simulink model "TST_EngPrt_PrtLimOvht"  (R2016b)
settings: Solver=FixedStepDiscrete  StartTime=0.0  StopTime=0.02  FixedStep=sampleTime  RelTol=1e-3
values from neighbouring files (symbols this model uses):
  testCase = 1    [initTST_EngPrt_PrtLimOvht_001.m]    (also in initTST_EngPrt_PrtLimOvht_002.m = 2; initTST_EngPrt_PrtLimOvht_003.m = 3; initTST_EngPrt_PrtLimOvht_004.m = 4; initTST_EngPrt_PrtLimOvht_005.m = 5)
libraries: simulink x21, UnitTest_Lib x10
(part 2 of 2)

== system TST_EngPrt_PrtLimOvht/simulationInput/testSignals_R003 ==
  BC : BusCreator  Inputs=14
  spec_AFS_mAirPerCyl : FromWorkspace  VariableName=testSig_AFS_mAirPerCyl  Interpolate=off  OutputAfterFinalValue=Holding final value
  spec_Air_tAFS_mp : FromWorkspace  VariableName=testSig_Air_tAFS_mp  Interpolate=off  OutputAfterFinalValue=Holding final value
  spec_Air_tCACDs_mp : FromWorkspace  VariableName=testSig_Air_tCACDs_mp  Interpolate=off  OutputAfterFinalValue=Holding final value
  spec_Air_tIntkVUs : FromWorkspace  VariableName=testSig_Air_tIntkVUs  Interpolate=off  OutputAfterFinalValue=Holding final value
  spec_CEngDsT_t : FromWorkspace  VariableName=testSig_CEngDsT_t  Interpolate=off  OutputAfterFinalValue=Holding final value
  spec_CnvSet_etaCurr : FromWorkspace  VariableName=testSig_CnvSet_etaCurr  Interpolate=off  OutputAfterFinalValue=Holding final value
  spec_DSM_bEngPrtOvhtPrv : FromWorkspace  VariableName=testSig_DSM_bEngPrtOvhtPrv  Interpolate=off  OutputAfterFinalValue=Holding final value
  spec_EngPrt_trqLimOvhtPrv : FromWorkspace  VariableName=testSig_EngPrt_trqLimOvhtPrv  Interpolate=off  OutputAfterFinalValue=Holding final value
  spec_EnvT_t : FromWorkspace  VariableName=testSig_EnvT_t  Interpolate=off  OutputAfterFinalValue=Holding final value
  spec_Epm_nEng : FromWorkspace  VariableName=testSig_Epm_nEng  Interpolate=off  OutputAfterFinalValue=Holding final value
  spec_FuelT_t : FromWorkspace  VariableName=testSig_FuelT_t  Interpolate=off  OutputAfterFinalValue=Holding final value
  spec_InjCtl_qSetUnBal : FromWorkspace  VariableName=testSig_InjCtl_qSetUnBal  Interpolate=off  OutputAfterFinalValue=Holding final value
  spec_Oil_tSwmp : FromWorkspace  VariableName=testSig_Oil_tSwmp  Interpolate=off  OutputAfterFinalValue=Holding final value
  spec_VehV_v : FromWorkspace  VariableName=testSig_VehV_v  Interpolate=off  OutputAfterFinalValue=Holding final value
  testSignals : Outport
  wires:
  BC/1 -> testSignals/1
  spec_Epm_nEng/1 -> BC/1  "testSig_Epm_nEng"
  spec_AFS_mAirPerCyl/1 -> BC/2  "testSig_AFS_mAirPerCyl"
  spec_InjCtl_qSetUnBal/1 -> BC/3  "testSig_InjCtl_qSetUnBal"
  spec_Oil_tSwmp/1 -> BC/4  "testSig_Oil_tSwmp"
  spec_CEngDsT_t/1 -> BC/5  "testSig_CEngDsT_t"
  spec_FuelT_t/1 -> BC/6  "testSig_FuelT_t"
  spec_VehV_v/1 -> BC/7  "testSig_VehV_v"
  spec_CnvSet_etaCurr/1 -> BC/8  "testSig_CnvSet_etaCurr"
  spec_DSM_bEngPrtOvhtPrv/1 -> BC/9  "testSig_DSM_bEngPrtOvhtPrv"
  spec_Air_tCACDs_mp/1 -> BC/10  "testSig_Air_tCACDs_mp"
  spec_Air_tAFS_mp/1 -> BC/11  "testSig_Air_tAFS_mp"
  spec_EnvT_t/1 -> BC/12  "testSig_EnvT_t"
  spec_Air_tIntkVUs/1 -> BC/13  "testSig_Air_tIntkVUs"
  spec_EngPrt_trqLimOvhtPrv/1 -> BC/14  "testSig_EngPrt_trqLimOvhtPrv"

== system TST_EngPrt_PrtLimOvht/simulationInput/testSignals_R004 ==
  BC : BusCreator  Inputs=14
  spec_AFS_mAirPerCyl : FromWorkspace  VariableName=testSig_AFS_mAirPerCyl  Interpolate=off  OutputAfterFinalValue=Holding final value
  spec_Air_tAFS_mp : FromWorkspace  VariableName=testSig_Air_tAFS_mp  Interpolate=off  OutputAfterFinalValue=Holding final value
  spec_Air_tCACDs_mp : FromWorkspace  VariableName=testSig_Air_tCACDs_mp  Interpolate=off  OutputAfterFinalValue=Holding final value
  spec_Air_tIntkVUs : FromWorkspace  VariableName=testSig_Air_tIntkVUs  Interpolate=off  OutputAfterFinalValue=Holding final value
  spec_CEngDsT_t : FromWorkspace  VariableName=testSig_CEngDsT_t  Interpolate=off  OutputAfterFinalValue=Holding final value
  spec_CnvSet_etaCurr : FromWorkspace  VariableName=testSig_CnvSet_etaCurr  Interpolate=off  OutputAfterFinalValue=Holding final value
  spec_DSM_bEngPrtOvhtPrv : FromWorkspace  VariableName=testSig_DSM_bEngPrtOvhtPrv  Interpolate=off  OutputAfterFinalValue=Holding final value
  spec_EngPrt_trqLimOvhtPrv : FromWorkspace  VariableName=testSig_EngPrt_trqLimOvhtPrv  Interpolate=off  OutputAfterFinalValue=Holding final value
  spec_EnvT_t : FromWorkspace  VariableName=testSig_EnvT_t  Interpolate=off  OutputAfterFinalValue=Holding final value
  spec_Epm_nEng : FromWorkspace  VariableName=testSig_Epm_nEng  Interpolate=off  OutputAfterFinalValue=Holding final value
  spec_FuelT_t : FromWorkspace  VariableName=testSig_FuelT_t  Interpolate=off  OutputAfterFinalValue=Holding final value
  spec_InjCtl_qSetUnBal : FromWorkspace  VariableName=testSig_InjCtl_qSetUnBal  Interpolate=off  OutputAfterFinalValue=Holding final value
  spec_Oil_tSwmp : FromWorkspace  VariableName=testSig_Oil_tSwmp  Interpolate=off  OutputAfterFinalValue=Holding final value
  spec_VehV_v : FromWorkspace  VariableName=testSig_VehV_v  Interpolate=off  OutputAfterFinalValue=Holding final value
  testSignals : Outport
  wires:
  BC/1 -> testSignals/1
  spec_Epm_nEng/1 -> BC/1  "testSig_Epm_nEng"
  spec_AFS_mAirPerCyl/1 -> BC/2  "testSig_AFS_mAirPerCyl"
  spec_InjCtl_qSetUnBal/1 -> BC/3  "testSig_InjCtl_qSetUnBal"
  spec_Oil_tSwmp/1 -> BC/4  "testSig_Oil_tSwmp"
  spec_CEngDsT_t/1 -> BC/5  "testSig_CEngDsT_t"
  spec_FuelT_t/1 -> BC/6  "testSig_FuelT_t"
  spec_VehV_v/1 -> BC/7  "testSig_VehV_v"
  spec_CnvSet_etaCurr/1 -> BC/8  "testSig_CnvSet_etaCurr"
  spec_DSM_bEngPrtOvhtPrv/1 -> BC/9  "testSig_DSM_bEngPrtOvhtPrv"
  spec_Air_tCACDs_mp/1 -> BC/10  "testSig_Air_tCACDs_mp"
  spec_Air_tAFS_mp/1 -> BC/11  "testSig_Air_tAFS_mp"
  spec_EnvT_t/1 -> BC/12  "testSig_EnvT_t"
  spec_Air_tIntkVUs/1 -> BC/13  "testSig_Air_tIntkVUs"
  spec_EngPrt_trqLimOvhtPrv/1 -> BC/14  "testSig_EngPrt_trqLimOvhtPrv"

== system TST_EngPrt_PrtLimOvht/simulationInput/testSignals_R005 ==
  BC : BusCreator  Inputs=14
  spec_AFS_mAirPerCyl : FromWorkspace  VariableName=testSig_AFS_mAirPerCyl  Interpolate=off  OutputAfterFinalValue=Holding final value
  spec_Air_tAFS_mp : FromWorkspace  VariableName=testSig_Air_tAFS_mp  Interpolate=off  OutputAfterFinalValue=Holding final value
  spec_Air_tCACDs_mp : FromWorkspace  VariableName=testSig_Air_tCACDs_mp  Interpolate=off  OutputAfterFinalValue=Holding final value
  spec_Air_tIntkVUs : FromWorkspace  VariableName=testSig_Air_tIntkVUs  Interpolate=off  OutputAfterFinalValue=Holding final value
  spec_CEngDsT_t : FromWorkspace  VariableName=testSig_CEngDsT_t  Interpolate=off  OutputAfterFinalValue=Holding final value
  spec_CnvSet_etaCurr : FromWorkspace  VariableName=testSig_CnvSet_etaCurr  Interpolate=off  OutputAfterFinalValue=Holding final value
  spec_DSM_bEngPrtOvhtPrv : FromWorkspace  VariableName=testSig_DSM_bEngPrtOvhtPrv  Interpolate=off  OutputAfterFinalValue=Holding final value
  spec_EngPrt_trqLimOvhtPrv : FromWorkspace  VariableName=testSig_EngPrt_trqLimOvhtPrv  Interpolate=off  OutputAfterFinalValue=Holding final value
  spec_EnvT_t : FromWorkspace  VariableName=testSig_EnvT_t  Interpolate=off  OutputAfterFinalValue=Holding final value
  spec_Epm_nEng : FromWorkspace  VariableName=testSig_Epm_nEng  Interpolate=off  OutputAfterFinalValue=Holding final value
  spec_FuelT_t : FromWorkspace  VariableName=testSig_FuelT_t  Interpolate=off  OutputAfterFinalValue=Holding final value
  spec_InjCtl_qSetUnBal : FromWorkspace  VariableName=testSig_InjCtl_qSetUnBal  Interpolate=off  OutputAfterFinalValue=Holding final value
  spec_Oil_tSwmp : FromWorkspace  VariableName=testSig_Oil_tSwmp  Interpolate=off  OutputAfterFinalValue=Holding final value
  spec_VehV_v : FromWorkspace  VariableName=testSig_VehV_v  Interpolate=off  OutputAfterFinalValue=Holding final value
  testSignals : Outport
  wires:
  BC/1 -> testSignals/1
  spec_Epm_nEng/1 -> BC/1  "testSig_Epm_nEng"
  spec_AFS_mAirPerCyl/1 -> BC/2  "testSig_AFS_mAirPerCyl"
  spec_InjCtl_qSetUnBal/1 -> BC/3  "testSig_InjCtl_qSetUnBal"
  spec_Oil_tSwmp/1 -> BC/4  "testSig_Oil_tSwmp"
  spec_CEngDsT_t/1 -> BC/5  "testSig_CEngDsT_t"
  spec_FuelT_t/1 -> BC/6  "testSig_FuelT_t"
  spec_VehV_v/1 -> BC/7  "testSig_VehV_v"
  spec_CnvSet_etaCurr/1 -> BC/8  "testSig_CnvSet_etaCurr"
  spec_DSM_bEngPrtOvhtPrv/1 -> BC/9  "testSig_DSM_bEngPrtOvhtPrv"
  spec_Air_tCACDs_mp/1 -> BC/10  "testSig_Air_tCACDs_mp"
  spec_Air_tAFS_mp/1 -> BC/11  "testSig_Air_tAFS_mp"
  spec_EnvT_t/1 -> BC/12  "testSig_EnvT_t"
  spec_Air_tIntkVUs/1 -> BC/13  "testSig_Air_tIntkVUs"
  spec_EngPrt_trqLimOvhtPrv/1 -> BC/14  "testSig_EngPrt_trqLimOvhtPrv"

== system TST_EngPrt_PrtLimOvht/simulationInput/testSignals_R006 ==
  BC : BusCreator  Inputs=14
  spec_AFS_mAirPerCyl : FromWorkspace  VariableName=testSig_AFS_mAirPerCyl  Interpolate=off  OutputAfterFinalValue=Holding final value
  spec_Air_tAFS_mp : FromWorkspace  VariableName=testSig_Air_tAFS_mp  Interpolate=off  OutputAfterFinalValue=Holding final value
  spec_Air_tCACDs_mp : FromWorkspace  VariableName=testSig_Air_tCACDs_mp  Interpolate=off  OutputAfterFinalValue=Holding final value
  spec_Air_tIntkVUs : FromWorkspace  VariableName=testSig_Air_tIntkVUs  Interpolate=off  OutputAfterFinalValue=Holding final value
  spec_CEngDsT_t : FromWorkspace  VariableName=testSig_CEngDsT_t  Interpolate=off  OutputAfterFinalValue=Holding final value
  spec_CnvSet_etaCurr : FromWorkspace  VariableName=testSig_CnvSet_etaCurr  Interpolate=off  OutputAfterFinalValue=Holding final value
  spec_DSM_bEngPrtOvhtPrv : FromWorkspace  VariableName=testSig_DSM_bEngPrtOvhtPrv  Interpolate=off  OutputAfterFinalValue=Holding final value
  spec_EngPrt_trqLimOvhtPrv : FromWorkspace  VariableName=testSig_EngPrt_trqLimOvhtPrv  Interpolate=off  OutputAfterFinalValue=Holding final value
  spec_EnvT_t : FromWorkspace  VariableName=testSig_EnvT_t  Interpolate=off  OutputAfterFinalValue=Holding final value
  spec_Epm_nEng : FromWorkspace  VariableName=testSig_Epm_nEng  Interpolate=off  OutputAfterFinalValue=Holding final value
  spec_FuelT_t : FromWorkspace  VariableName=testSig_FuelT_t  Interpolate=off  OutputAfterFinalValue=Holding final value
  spec_InjCtl_qSetUnBal : FromWorkspace  VariableName=testSig_InjCtl_qSetUnBal  Interpolate=off  OutputAfterFinalValue=Holding final value
  spec_Oil_tSwmp : FromWorkspace  VariableName=testSig_Oil_tSwmp  Interpolate=off  OutputAfterFinalValue=Holding final value
  spec_VehV_v : FromWorkspace  VariableName=testSig_VehV_v  Interpolate=off  OutputAfterFinalValue=Holding final value
  testSignals : Outport
  wires:
  BC/1 -> testSignals/1
  spec_Epm_nEng/1 -> BC/1  "testSig_Epm_nEng"
  spec_AFS_mAirPerCyl/1 -> BC/2  "testSig_AFS_mAirPerCyl"
  spec_InjCtl_qSetUnBal/1 -> BC/3  "testSig_InjCtl_qSetUnBal"
  spec_Oil_tSwmp/1 -> BC/4  "testSig_Oil_tSwmp"
  spec_CEngDsT_t/1 -> BC/5  "testSig_CEngDsT_t"
  spec_FuelT_t/1 -> BC/6  "testSig_FuelT_t"
  spec_VehV_v/1 -> BC/7  "testSig_VehV_v"
  spec_CnvSet_etaCurr/1 -> BC/8  "testSig_CnvSet_etaCurr"
  spec_DSM_bEngPrtOvhtPrv/1 -> BC/9  "testSig_DSM_bEngPrtOvhtPrv"
  spec_Air_tCACDs_mp/1 -> BC/10  "testSig_Air_tCACDs_mp"
  spec_Air_tAFS_mp/1 -> BC/11  "testSig_Air_tAFS_mp"
  spec_EnvT_t/1 -> BC/12  "testSig_EnvT_t"
  spec_Air_tIntkVUs/1 -> BC/13  "testSig_Air_tIntkVUs"
  spec_EngPrt_trqLimOvhtPrv/1 -> BC/14  "testSig_EngPrt_trqLimOvhtPrv"

== system TST_EngPrt_PrtLimOvht/simulationInput/testSignals_R007 ==
  BC : BusCreator  Inputs=14
  spec_AFS_mAirPerCyl : FromWorkspace  VariableName=testSig_AFS_mAirPerCyl  Interpolate=off  OutputAfterFinalValue=Holding final value
  spec_Air_tAFS_mp : FromWorkspace  VariableName=testSig_Air_tAFS_mp  Interpolate=off  OutputAfterFinalValue=Holding final value
  spec_Air_tCACDs_mp : FromWorkspace  VariableName=testSig_Air_tCACDs_mp  Interpolate=off  OutputAfterFinalValue=Holding final value
  spec_Air_tIntkVUs : FromWorkspace  VariableName=testSig_Air_tIntkVUs  Interpolate=off  OutputAfterFinalValue=Holding final value
  spec_CEngDsT_t : FromWorkspace  VariableName=testSig_CEngDsT_t  Interpolate=off  OutputAfterFinalValue=Holding final value
  spec_CnvSet_etaCurr : FromWorkspace  VariableName=testSig_CnvSet_etaCurr  Interpolate=off  OutputAfterFinalValue=Holding final value
  spec_DSM_bEngPrtOvhtPrv : FromWorkspace  VariableName=testSig_DSM_bEngPrtOvhtPrv  Interpolate=off  OutputAfterFinalValue=Holding final value
  spec_EngPrt_trqLimOvhtPrv : FromWorkspace  VariableName=testSig_EngPrt_trqLimOvhtPrv  Interpolate=off  OutputAfterFinalValue=Holding final value
  spec_EnvT_t : FromWorkspace  VariableName=testSig_EnvT_t  Interpolate=off  OutputAfterFinalValue=Holding final value
  spec_Epm_nEng : FromWorkspace  VariableName=testSig_Epm_nEng  Interpolate=off  OutputAfterFinalValue=Holding final value
  spec_FuelT_t : FromWorkspace  VariableName=testSig_FuelT_t  Interpolate=off  OutputAfterFinalValue=Holding final value
  spec_InjCtl_qSetUnBal : FromWorkspace  VariableName=testSig_InjCtl_qSetUnBal  Interpolate=off  OutputAfterFinalValue=Holding final value
  spec_Oil_tSwmp : FromWorkspace  VariableName=testSig_Oil_tSwmp  Interpolate=off  OutputAfterFinalValue=Holding final value
  spec_VehV_v : FromWorkspace  VariableName=testSig_VehV_v  Interpolate=off  OutputAfterFinalValue=Holding final value
  testSignals : Outport
  wires:
  BC/1 -> testSignals/1
  spec_Epm_nEng/1 -> BC/1  "testSig_Epm_nEng"
  spec_AFS_mAirPerCyl/1 -> BC/2  "testSig_AFS_mAirPerCyl"
  spec_InjCtl_qSetUnBal/1 -> BC/3  "testSig_InjCtl_qSetUnBal"
  spec_Oil_tSwmp/1 -> BC/4  "testSig_Oil_tSwmp"
  spec_CEngDsT_t/1 -> BC/5  "testSig_CEngDsT_t"
  spec_FuelT_t/1 -> BC/6  "testSig_FuelT_t"
  spec_VehV_v/1 -> BC/7  "testSig_VehV_v"
  spec_CnvSet_etaCurr/1 -> BC/8  "testSig_CnvSet_etaCurr"
  spec_DSM_bEngPrtOvhtPrv/1 -> BC/9  "testSig_DSM_bEngPrtOvhtPrv"
  spec_Air_tCACDs_mp/1 -> BC/10  "testSig_Air_tCACDs_mp"
  spec_Air_tAFS_mp/1 -> BC/11  "testSig_Air_tAFS_mp"
  spec_EnvT_t/1 -> BC/12  "testSig_EnvT_t"
  spec_Air_tIntkVUs/1 -> BC/13  "testSig_Air_tIntkVUs"
  spec_EngPrt_trqLimOvhtPrv/1 -> BC/14  "testSig_EngPrt_trqLimOvhtPrv"

== system TST_EngPrt_PrtLimOvht/simulationInput/testSignals_R008 ==
  BC : BusCreator  Inputs=14
  spec_AFS_mAirPerCyl : FromWorkspace  VariableName=testSig_AFS_mAirPerCyl  Interpolate=off  OutputAfterFinalValue=Holding final value
  spec_Air_tAFS_mp : FromWorkspace  VariableName=testSig_Air_tAFS_mp  Interpolate=off  OutputAfterFinalValue=Holding final value
  spec_Air_tCACDs_mp : FromWorkspace  VariableName=testSig_Air_tCACDs_mp  Interpolate=off  OutputAfterFinalValue=Holding final value
  spec_Air_tIntkVUs : FromWorkspace  VariableName=testSig_Air_tIntkVUs  Interpolate=off  OutputAfterFinalValue=Holding final value
  spec_CEngDsT_t : FromWorkspace  VariableName=testSig_CEngDsT_t  Interpolate=off  OutputAfterFinalValue=Holding final value
  spec_CnvSet_etaCurr : FromWorkspace  VariableName=testSig_CnvSet_etaCurr  Interpolate=off  OutputAfterFinalValue=Holding final value
  spec_DSM_bEngPrtOvhtPrv : FromWorkspace  VariableName=testSig_DSM_bEngPrtOvhtPrv  Interpolate=off  OutputAfterFinalValue=Holding final value
  spec_EngPrt_trqLimOvhtPrv : FromWorkspace  VariableName=testSig_EngPrt_trqLimOvhtPrv  Interpolate=off  OutputAfterFinalValue=Holding final value
  spec_EnvT_t : FromWorkspace  VariableName=testSig_EnvT_t  Interpolate=off  OutputAfterFinalValue=Holding final value
  spec_Epm_nEng : FromWorkspace  VariableName=testSig_Epm_nEng  Interpolate=off  OutputAfterFinalValue=Holding final value
  spec_FuelT_t : FromWorkspace  VariableName=testSig_FuelT_t  Interpolate=off  OutputAfterFinalValue=Holding final value
  spec_InjCtl_qSetUnBal : FromWorkspace  VariableName=testSig_InjCtl_qSetUnBal  Interpolate=off  OutputAfterFinalValue=Holding final value
  spec_Oil_tSwmp : FromWorkspace  VariableName=testSig_Oil_tSwmp  Interpolate=off  OutputAfterFinalValue=Holding final value
  spec_VehV_v : FromWorkspace  VariableName=testSig_VehV_v  Interpolate=off  OutputAfterFinalValue=Holding final value
  testSignals : Outport
  wires:
  BC/1 -> testSignals/1
  spec_Epm_nEng/1 -> BC/1  "testSig_Epm_nEng"
  spec_AFS_mAirPerCyl/1 -> BC/2  "testSig_AFS_mAirPerCyl"
  spec_InjCtl_qSetUnBal/1 -> BC/3  "testSig_InjCtl_qSetUnBal"
  spec_Oil_tSwmp/1 -> BC/4  "testSig_Oil_tSwmp"
  spec_CEngDsT_t/1 -> BC/5  "testSig_CEngDsT_t"
  spec_FuelT_t/1 -> BC/6  "testSig_FuelT_t"
  spec_VehV_v/1 -> BC/7  "testSig_VehV_v"
  spec_CnvSet_etaCurr/1 -> BC/8  "testSig_CnvSet_etaCurr"
  spec_DSM_bEngPrtOvhtPrv/1 -> BC/9  "testSig_DSM_bEngPrtOvhtPrv"
  spec_Air_tCACDs_mp/1 -> BC/10  "testSig_Air_tCACDs_mp"
  spec_Air_tAFS_mp/1 -> BC/11  "testSig_Air_tAFS_mp"
  spec_EnvT_t/1 -> BC/12  "testSig_EnvT_t"
  spec_Air_tIntkVUs/1 -> BC/13  "testSig_Air_tIntkVUs"
  spec_EngPrt_trqLimOvhtPrv/1 -> BC/14  "testSig_EngPrt_trqLimOvhtPrv"

== system TST_EngPrt_PrtLimOvht/simulationInput/testSignals_R009 ==
  BC : BusCreator  Inputs=14
  spec_AFS_mAirPerCyl : FromWorkspace  VariableName=testSig_AFS_mAirPerCyl  Interpolate=off  OutputAfterFinalValue=Holding final value
  spec_Air_tAFS_mp : FromWorkspace  VariableName=testSig_Air_tAFS_mp  Interpolate=off  OutputAfterFinalValue=Holding final value
  spec_Air_tCACDs_mp : FromWorkspace  VariableName=testSig_Air_tCACDs_mp  Interpolate=off  OutputAfterFinalValue=Holding final value
  spec_Air_tIntkVUs : FromWorkspace  VariableName=testSig_Air_tIntkVUs  Interpolate=off  OutputAfterFinalValue=Holding final value
  spec_CEngDsT_t : FromWorkspace  VariableName=testSig_CEngDsT_t  Interpolate=off  OutputAfterFinalValue=Holding final value
  spec_CnvSet_etaCurr : FromWorkspace  VariableName=testSig_CnvSet_etaCurr  Interpolate=off  OutputAfterFinalValue=Holding final value
  spec_DSM_bEngPrtOvhtPrv : FromWorkspace  VariableName=testSig_DSM_bEngPrtOvhtPrv  Interpolate=off  OutputAfterFinalValue=Holding final value
  spec_EngPrt_trqLimOvhtPrv : FromWorkspace  VariableName=testSig_EngPrt_trqLimOvhtPrv  Interpolate=off  OutputAfterFinalValue=Holding final value
  spec_EnvT_t : FromWorkspace  VariableName=testSig_EnvT_t  Interpolate=off  OutputAfterFinalValue=Holding final value
  spec_Epm_nEng : FromWorkspace  VariableName=testSig_Epm_nEng  Interpolate=off  OutputAfterFinalValue=Holding final value
  spec_FuelT_t : FromWorkspace  VariableName=testSig_FuelT_t  Interpolate=off  OutputAfterFinalValue=Holding final value
  spec_InjCtl_qSetUnBal : FromWorkspace  VariableName=testSig_InjCtl_qSetUnBal  Interpolate=off  OutputAfterFinalValue=Holding final value
  spec_Oil_tSwmp : FromWorkspace  VariableName=testSig_Oil_tSwmp  Interpolate=off  OutputAfterFinalValue=Holding final value
  spec_VehV_v : FromWorkspace  VariableName=testSig_VehV_v  Interpolate=off  OutputAfterFinalValue=Holding final value
  testSignals : Outport
  wires:
  BC/1 -> testSignals/1
  spec_Epm_nEng/1 -> BC/1  "testSig_Epm_nEng"
  spec_AFS_mAirPerCyl/1 -> BC/2  "testSig_AFS_mAirPerCyl"
  spec_InjCtl_qSetUnBal/1 -> BC/3  "testSig_InjCtl_qSetUnBal"
  spec_Oil_tSwmp/1 -> BC/4  "testSig_Oil_tSwmp"
  spec_CEngDsT_t/1 -> BC/5  "testSig_CEngDsT_t"
  spec_FuelT_t/1 -> BC/6  "testSig_FuelT_t"
  spec_VehV_v/1 -> BC/7  "testSig_VehV_v"
  spec_CnvSet_etaCurr/1 -> BC/8  "testSig_CnvSet_etaCurr"
  spec_DSM_bEngPrtOvhtPrv/1 -> BC/9  "testSig_DSM_bEngPrtOvhtPrv"
  spec_Air_tCACDs_mp/1 -> BC/10  "testSig_Air_tCACDs_mp"
  spec_Air_tAFS_mp/1 -> BC/11  "testSig_Air_tAFS_mp"
  spec_EnvT_t/1 -> BC/12  "testSig_EnvT_t"
  spec_Air_tIntkVUs/1 -> BC/13  "testSig_Air_tIntkVUs"
  spec_EngPrt_trqLimOvhtPrv/1 -> BC/14  "testSig_EngPrt_trqLimOvhtPrv"

== system TST_EngPrt_PrtLimOvht/simulationInput/testSignals_R010 ==
  BC : BusCreator  Inputs=14
  spec_AFS_mAirPerCyl : FromWorkspace  VariableName=testSig_AFS_mAirPerCyl  Interpolate=off  OutputAfterFinalValue=Holding final value
  spec_Air_tAFS_mp : FromWorkspace  VariableName=testSig_Air_tAFS_mp  Interpolate=off  OutputAfterFinalValue=Holding final value
  spec_Air_tCACDs_mp : FromWorkspace  VariableName=testSig_Air_tCACDs_mp  Interpolate=off  OutputAfterFinalValue=Holding final value
  spec_Air_tIntkVUs : FromWorkspace  VariableName=testSig_Air_tIntkVUs  Interpolate=off  OutputAfterFinalValue=Holding final value
  spec_CEngDsT_t : FromWorkspace  VariableName=testSig_CEngDsT_t  Interpolate=off  OutputAfterFinalValue=Holding final value
  spec_CnvSet_etaCurr : FromWorkspace  VariableName=testSig_CnvSet_etaCurr  Interpolate=off  OutputAfterFinalValue=Holding final value
  spec_DSM_bEngPrtOvhtPrv : FromWorkspace  VariableName=testSig_DSM_bEngPrtOvhtPrv  Interpolate=off  OutputAfterFinalValue=Holding final value
  spec_EngPrt_trqLimOvhtPrv : FromWorkspace  VariableName=testSig_EngPrt_trqLimOvhtPrv  Interpolate=off  OutputAfterFinalValue=Holding final value
  spec_EnvT_t : FromWorkspace  VariableName=testSig_EnvT_t  Interpolate=off  OutputAfterFinalValue=Holding final value
  spec_Epm_nEng : FromWorkspace  VariableName=testSig_Epm_nEng  Interpolate=off  OutputAfterFinalValue=Holding final value
  spec_FuelT_t : FromWorkspace  VariableName=testSig_FuelT_t  Interpolate=off  OutputAfterFinalValue=Holding final value
  spec_InjCtl_qSetUnBal : FromWorkspace  VariableName=testSig_InjCtl_qSetUnBal  Interpolate=off  OutputAfterFinalValue=Holding final value
  spec_Oil_tSwmp : FromWorkspace  VariableName=testSig_Oil_tSwmp  Interpolate=off  OutputAfterFinalValue=Holding final value
  spec_VehV_v : FromWorkspace  VariableName=testSig_VehV_v  Interpolate=off  OutputAfterFinalValue=Holding final value
  testSignals : Outport
  wires:
  BC/1 -> testSignals/1
  spec_Epm_nEng/1 -> BC/1  "testSig_Epm_nEng"
  spec_AFS_mAirPerCyl/1 -> BC/2  "testSig_AFS_mAirPerCyl"
  spec_InjCtl_qSetUnBal/1 -> BC/3  "testSig_InjCtl_qSetUnBal"
  spec_Oil_tSwmp/1 -> BC/4  "testSig_Oil_tSwmp"
  spec_CEngDsT_t/1 -> BC/5  "testSig_CEngDsT_t"
  spec_FuelT_t/1 -> BC/6  "testSig_FuelT_t"
  spec_VehV_v/1 -> BC/7  "testSig_VehV_v"
  spec_CnvSet_etaCurr/1 -> BC/8  "testSig_CnvSet_etaCurr"
  spec_DSM_bEngPrtOvhtPrv/1 -> BC/9  "testSig_DSM_bEngPrtOvhtPrv"
  spec_Air_tCACDs_mp/1 -> BC/10  "testSig_Air_tCACDs_mp"
  spec_Air_tAFS_mp/1 -> BC/11  "testSig_Air_tAFS_mp"
  spec_EnvT_t/1 -> BC/12  "testSig_EnvT_t"
  spec_Air_tIntkVUs/1 -> BC/13  "testSig_Air_tIntkVUs"
  spec_EngPrt_trqLimOvhtPrv/1 -> BC/14  "testSig_EngPrt_trqLimOvhtPrv"

== system TST_EngPrt_PrtLimOvht/compareSignals/Requirement_001/specifyOutputs ==
  sig_Req_Bus : Inport
  sig_Result_Bus : Inport  Port=2
  AndN : Logic  Inputs=1
  BS_Req : BusSelector  OutputSignals=testSig_EngPrt_trqLimOvhtPrv
  BS_Result : BusSelector  OutputSignals=EngPrt_trqLimOvhtPrv
  Bitwise_And1 : simulink/Logic and Bit Operations/Bitwise Operator  logicop=AND  UseBitMask=off  BitMask=bin2dec('11011001')  BitMaskRealWorld=Stored Integer
  Scope : Scope
  Scope1 : Scope  NumInputPorts=2
  cmp_1 : UnitTest_Lib/RoughlyEqual  slope=0.1
  result_tws : ToWorkspace  VariableName=spec_result_001
  tws_1 : ToWorkspace  VariableName=spec_req_001_001
  result : Outport
  wires:
  sig_Req_Bus/1 -> BS_Req/1
  sig_Result_Bus/1 -> BS_Result/1
  AndN/1 -> result/1, result_tws/1
  BS_Req/1 -> cmp_1/1, Scope1/1  "<testSig_EngPrt_trqLimOvhtPrv>"
  BS_Result/1 -> cmp_1/2, Scope1/2  "<EngPrt_trqLimOvhtPrv>"
  cmp_1/1 -> Bitwise_And1/1
  Bitwise_And1/1 -> tws_1/1, AndN/1, Scope/1

== system TST_EngPrt_PrtLimOvht/compareSignals/Requirement_002/specifyOutputs ==
  sig_Req_Bus : Inport
  sig_Result_Bus : Inport  Port=2
  AndN : Logic  Inputs=1
  BS_Req : BusSelector  OutputSignals=testSig_EngPrt_trqLimOvhtPrv
  BS_Result : BusSelector  OutputSignals=EngPrt_trqLimOvhtPrv
  Bitwise_And1 : simulink/Logic and Bit Operations/Bitwise Operator  logicop=AND  UseBitMask=off  BitMask=bin2dec('11011001')  BitMaskRealWorld=Stored Integer
  Scope : Scope
  Scope1 : Scope  NumInputPorts=2
  cmp_1 : UnitTest_Lib/RoughlyEqual  slope=0.1
  result_tws : ToWorkspace  VariableName=spec_result_002
  tws_1 : ToWorkspace  VariableName=spec_req_002_001
  result : Outport
  wires:
  sig_Req_Bus/1 -> BS_Req/1
  sig_Result_Bus/1 -> BS_Result/1
  AndN/1 -> result/1, result_tws/1
  BS_Req/1 -> cmp_1/1, Scope1/1  "<testSig_EngPrt_trqLimOvhtPrv>"
  BS_Result/1 -> cmp_1/2, Scope1/2  "<EngPrt_trqLimOvhtPrv>"
  cmp_1/1 -> Bitwise_And1/1
  Bitwise_And1/1 -> tws_1/1, AndN/1, Scope/1

== system TST_EngPrt_PrtLimOvht/compareSignals/Requirement_003/specifyOutputs ==
  sig_Req_Bus : Inport
  sig_Result_Bus : Inport  Port=2
  AndN : Logic  Inputs=1
  BS_Req : BusSelector  OutputSignals=testSig_EngPrt_trqLimOvhtPrv
  BS_Result : BusSelector  OutputSignals=EngPrt_trqLimOvhtPrv
  Bitwise_And1 : simulink/Logic and Bit Operations/Bitwise Operator  logicop=AND  UseBitMask=off  BitMask=bin2dec('11011001')  BitMaskRealWorld=Stored Integer
  Scope : Scope
  Scope1 : Scope  NumInputPorts=2
  cmp_1 : UnitTest_Lib/RoughlyEqual  slope=0.1
  result_tws : ToWorkspace  VariableName=spec_result_003
  tws_1 : ToWorkspace  VariableName=spec_req_003_001
  result : Outport
  wires:
  sig_Req_Bus/1 -> BS_Req/1
  sig_Result_Bus/1 -> BS_Result/1
  AndN/1 -> result/1, result_tws/1
  BS_Req/1 -> cmp_1/1, Scope1/1  "<testSig_EngPrt_trqLimOvhtPrv>"
  BS_Result/1 -> cmp_1/2, Scope1/2  "<EngPrt_trqLimOvhtPrv>"
  cmp_1/1 -> Bitwise_And1/1
  Bitwise_And1/1 -> AndN/1, Scope/1, tws_1/1

== system TST_EngPrt_PrtLimOvht/compareSignals/Requirement_004/specifyOutputs ==
  sig_Req_Bus : Inport
  sig_Result_Bus : Inport  Port=2
  AndN : Logic  Inputs=1
  BS_Req : BusSelector  OutputSignals=testSig_EngPrt_trqLimOvhtPrv
  BS_Result : BusSelector  OutputSignals=EngPrt_trqLimOvhtPrv
  Bitwise_And1 : simulink/Logic and Bit Operations/Bitwise Operator  logicop=AND  UseBitMask=off  BitMask=bin2dec('11011001')  BitMaskRealWorld=Stored Integer
  Scope : Scope
  Scope1 : Scope  NumInputPorts=2
  cmp_1 : UnitTest_Lib/RoughlyEqual  slope=0.5
  result_tws : ToWorkspace  VariableName=spec_result_004
  tws_1 : ToWorkspace  VariableName=spec_req_004_001
  result : Outport
  wires:
  sig_Req_Bus/1 -> BS_Req/1
  sig_Result_Bus/1 -> BS_Result/1
  AndN/1 -> result/1, result_tws/1
  BS_Req/1 -> cmp_1/1, Scope1/1  "<testSig_EngPrt_trqLimOvhtPrv>"
  BS_Result/1 -> cmp_1/2, Scope1/2  "<EngPrt_trqLimOvhtPrv>"
  cmp_1/1 -> Bitwise_And1/1
  Bitwise_And1/1 -> AndN/1, Scope/1, tws_1/1

== system TST_EngPrt_PrtLimOvht/compareSignals/Requirement_005/specifyOutputs ==
  sig_Req_Bus : Inport
  sig_Result_Bus : Inport  Port=2
  AndN : Logic  Inputs=1
  BS_Req : BusSelector  OutputSignals=testSig_EngPrt_trqLimOvhtPrv
  BS_Result : BusSelector  OutputSignals=EngPrt_trqLimOvhtPrv
  Bitwise_And1 : simulink/Logic and Bit Operations/Bitwise Operator  logicop=AND  UseBitMask=off  BitMask=bin2dec('11011001')  BitMaskRealWorld=Stored Integer
  Scope : Scope
  Scope1 : Scope  NumInputPorts=2
  cmp_1 : UnitTest_Lib/RoughlyEqual  slope=0.5
  result_tws : ToWorkspace  VariableName=spec_result_005
  tws_1 : ToWorkspace  VariableName=spec_req_005_001
  result : Outport
  wires:
  sig_Req_Bus/1 -> BS_Req/1
  sig_Result_Bus/1 -> BS_Result/1
  AndN/1 -> result/1, result_tws/1
  BS_Req/1 -> cmp_1/1, Scope1/1  "<testSig_EngPrt_trqLimOvhtPrv>"
  BS_Result/1 -> cmp_1/2, Scope1/2  "<EngPrt_trqLimOvhtPrv>"
  cmp_1/1 -> Bitwise_And1/1
  Bitwise_And1/1 -> AndN/1, Scope/1, tws_1/1

== system TST_EngPrt_PrtLimOvht/compareSignals/Requirement_006/specifyOutputs ==
  sig_Req_Bus : Inport
  sig_Result_Bus : Inport  Port=2
  AndN : Logic  Inputs=1
  BS_Req : BusSelector  OutputSignals=testSig_EngPrt_trqLimOvhtPrv
  BS_Result : BusSelector  OutputSignals=EngPrt_trqLimOvhtPrv
  Bitwise_And1 : simulink/Logic and Bit Operations/Bitwise Operator  logicop=AND  UseBitMask=off  BitMask=bin2dec('11011001')  BitMaskRealWorld=Stored Integer
  Scope : Scope
  Scope1 : Scope  NumInputPorts=2
  cmp_1 : UnitTest_Lib/RoughlyEqual  slope=0.5
  result_tws : ToWorkspace  VariableName=spec_result_006
  tws_1 : ToWorkspace  VariableName=spec_req_006_001
  result : Outport
  wires:
  sig_Req_Bus/1 -> BS_Req/1
  sig_Result_Bus/1 -> BS_Result/1
  AndN/1 -> result/1, result_tws/1
  BS_Req/1 -> cmp_1/1, Scope1/1  "<testSig_EngPrt_trqLimOvhtPrv>"
  BS_Result/1 -> cmp_1/2, Scope1/2  "<EngPrt_trqLimOvhtPrv>"
  cmp_1/1 -> Bitwise_And1/1
  Bitwise_And1/1 -> AndN/1, Scope/1, tws_1/1

== system TST_EngPrt_PrtLimOvht/compareSignals/Requirement_007/specifyOutputs ==
  sig_Req_Bus : Inport
  sig_Result_Bus : Inport  Port=2
  AndN : Logic  Inputs=1
  BS_Req : BusSelector  OutputSignals=testSig_EngPrt_trqLimOvhtPrv
  BS_Result : BusSelector  OutputSignals=EngPrt_trqLimOvhtPrv
  Bitwise_And1 : simulink/Logic and Bit Operations/Bitwise Operator  logicop=AND  UseBitMask=off  BitMask=bin2dec('11011001')  BitMaskRealWorld=Stored Integer
  Scope : Scope
  Scope1 : Scope  NumInputPorts=2
  cmp_1 : UnitTest_Lib/RoughlyEqual  slope=0.5
  result_tws : ToWorkspace  VariableName=spec_result_007
  tws_1 : ToWorkspace  VariableName=spec_req_007_001
  result : Outport
  wires:
  sig_Req_Bus/1 -> BS_Req/1
  sig_Result_Bus/1 -> BS_Result/1
  AndN/1 -> result/1, result_tws/1
  BS_Req/1 -> cmp_1/1, Scope1/1  "<testSig_EngPrt_trqLimOvhtPrv>"
  BS_Result/1 -> cmp_1/2, Scope1/2  "<EngPrt_trqLimOvhtPrv>"
  cmp_1/1 -> Bitwise_And1/1
  Bitwise_And1/1 -> AndN/1, Scope/1, tws_1/1

== system TST_EngPrt_PrtLimOvht/compareSignals/Requirement_008/specifyOutputs ==
  sig_Req_Bus : Inport
  sig_Result_Bus : Inport  Port=2
  AndN : Logic  Inputs=1
  BS_Req : BusSelector  OutputSignals=testSig_EngPrt_trqLimOvhtPrv
  BS_Result : BusSelector  OutputSignals=EngPrt_trqLimOvhtPrv
  Bitwise_And1 : simulink/Logic and Bit Operations/Bitwise Operator  logicop=AND  UseBitMask=off  BitMask=bin2dec('11011001')  BitMaskRealWorld=Stored Integer
  Scope : Scope
  Scope1 : Scope  NumInputPorts=2
  cmp_1 : UnitTest_Lib/RoughlyEqual  slope=0.1
  result_tws : ToWorkspace  VariableName=spec_result_008
  tws_1 : ToWorkspace  VariableName=spec_req_008_001
  result : Outport
  wires:
  sig_Req_Bus/1 -> BS_Req/1
  sig_Result_Bus/1 -> BS_Result/1
  AndN/1 -> result/1, result_tws/1
  BS_Req/1 -> cmp_1/1, Scope1/1  "<testSig_EngPrt_trqLimOvhtPrv>"
  BS_Result/1 -> cmp_1/2, Scope1/2  "<EngPrt_trqLimOvhtPrv>"
  cmp_1/1 -> Bitwise_And1/1
  Bitwise_And1/1 -> tws_1/1, AndN/1, Scope/1

== system TST_EngPrt_PrtLimOvht/compareSignals/Requirement_009/specifyOutputs ==
  sig_Req_Bus : Inport
  sig_Result_Bus : Inport  Port=2
  AndN : Logic  Inputs=1
  BS_Req : BusSelector  OutputSignals=testSig_EngPrt_trqLimOvhtPrv
  BS_Result : BusSelector  OutputSignals=EngPrt_trqLimOvhtPrv
  Bitwise_And1 : simulink/Logic and Bit Operations/Bitwise Operator  logicop=AND  UseBitMask=off  BitMask=bin2dec('11011001')  BitMaskRealWorld=Stored Integer
  Scope : Scope
  Scope1 : Scope  NumInputPorts=2
  cmp_1 : UnitTest_Lib/RoughlyEqual  slope=0.1
  result_tws : ToWorkspace  VariableName=spec_result_009
  tws_1 : ToWorkspace  VariableName=spec_req_009_001
  result : Outport
  wires:
  sig_Req_Bus/1 -> BS_Req/1
  sig_Result_Bus/1 -> BS_Result/1
  AndN/1 -> result/1, result_tws/1
  BS_Req/1 -> cmp_1/1, Scope1/1  "<testSig_EngPrt_trqLimOvhtPrv>"
  BS_Result/1 -> cmp_1/2, Scope1/2  "<EngPrt_trqLimOvhtPrv>"
  cmp_1/1 -> Bitwise_And1/1
  Bitwise_And1/1 -> tws_1/1, AndN/1, Scope/1

== system TST_EngPrt_PrtLimOvht/compareSignals/Requirement_010/specifyOutputs ==
  sig_Req_Bus : Inport
  sig_Result_Bus : Inport  Port=2
  AndN : Logic  Inputs=1
  BS_Req : BusSelector  OutputSignals=testSig_EngPrt_trqLimOvhtPrv
  BS_Result : BusSelector  OutputSignals=EngPrt_trqLimOvhtPrv
  Bitwise_And1 : simulink/Logic and Bit Operations/Bitwise Operator  logicop=AND  UseBitMask=off  BitMask=bin2dec('11011001')  BitMaskRealWorld=Stored Integer
  Scope : Scope
  Scope1 : Scope  NumInputPorts=2
  cmp_1 : UnitTest_Lib/RoughlyEqual  slope=0.1
  result_tws : ToWorkspace  VariableName=spec_result_010
  tws_1 : ToWorkspace  VariableName=spec_req_010_001
  result : Outport
  wires:
  sig_Req_Bus/1 -> BS_Req/1
  sig_Result_Bus/1 -> BS_Result/1
  AndN/1 -> result/1, result_tws/1
  BS_Req/1 -> cmp_1/1, Scope1/1  "<testSig_EngPrt_trqLimOvhtPrv>"
  BS_Result/1 -> cmp_1/2, Scope1/2  "<EngPrt_trqLimOvhtPrv>"
  cmp_1/1 -> Bitwise_And1/1
  Bitwise_And1/1 -> tws_1/1, AndN/1, Scope/1
